simulink model "ME561FinalProjectSimulink_DiscreteNoFbOptimized_Stability"  (R2020a)
settings: Solver=ode5  StartTime=0.0  StopTime=800  FixedStep=0.01  RelTol=1e-3
values from neighbouring files (symbols this model uses):
  dB = 0.87    [ME561FinalProject.m]
  g = -9.81    [ME561FinalProject.m]
  humanSamplingTime = 0.01    [ME561FinalProject.m]
  JB = 66    [ME561FinalProject.m]
  KdDiscrete = K*Td/T    (= 19500)    [ME561FinalProject.m]
  KiDiscrete = K*T/Ti    (= 30)    [ME561FinalProject.m]
  Kn = 462    [ME561FinalProject.m]
  KpDiscrete = K - K*T/(2*Ti)    (= 435)    [ME561FinalProject.m]
  mB = 76    [ME561FinalProject.m]
  thetaRef = 0    [ME561FinalProject.m]
  timeNoise = 100    [ME561FinalProject.m]
libraries: simulink x1, simulink_extras x1
settings Model: Creator=jcferris  LastModifiedBy=jcferris

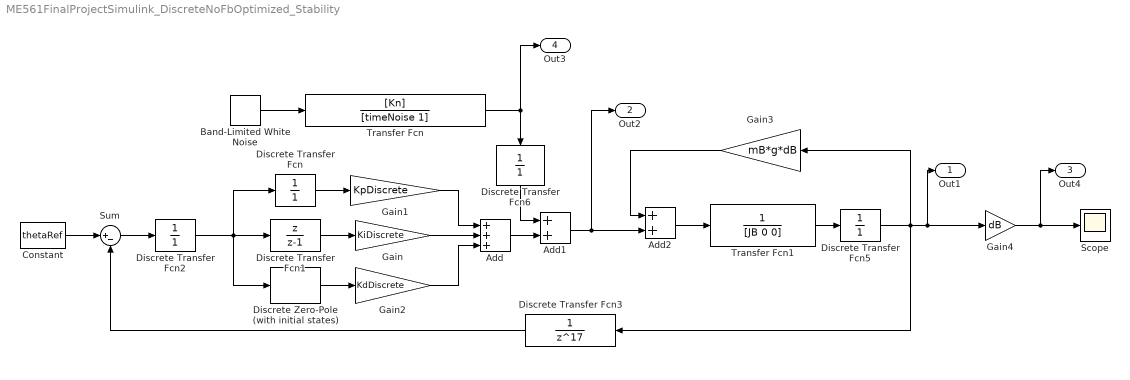
== system ME561FinalProjectSimulink_DiscreteNoFbOptimized_Stability ==
  Add : Sum  Inputs=+++
  Add1 : Sum
  Add2 : Sum
  Band-Limited White Noise : simulink/Sources/Band-Limited White Noise  Cov=[0.01]  Ts=0.01  seed=[23341]
  Constant : Constant  Value=thetaRef
  Discrete Transfer Fcn : DiscreteTransferFcn  Denominator=[1]
  Discrete Transfer Fcn1 : DiscreteTransferFcn  Numerator=[1 0]  Denominator=[1 -1]
  Discrete Transfer Fcn2 : DiscreteTransferFcn  Denominator=[1]  SampleTime=humanSamplingTime
  Discrete Transfer Fcn3 : DiscreteTransferFcn  Denominator=[1 0 0 0 0 0 0 0 0 0 0 0 0 0 0 0 0 0]
  Discrete Transfer Fcn5 : DiscreteTransferFcn  Denominator=[1]  SampleTime=humanSamplingTime
  Discrete Transfer Fcn6 : DiscreteTransferFcn  Denominator=[1]  SampleTime=humanSamplingTime
  Discrete Zero-Pole (with initial states) : simulink_extras/Additional Discrete/Discrete Zero-Pole (with initial states)  Z=[1]  P=[0]  K=[1]  X0=0  TS=-1
      settings: SourceProductBaseCode=SL
  Gain : Gain  Gain=KiDiscrete
  Gain1 : Gain  Gain=KpDiscrete
  Gain2 : Gain  Gain=KdDiscrete
  Gain3 : Gain  Gain=mB*g*dB
  Gain4 : Gain  Gain=dB
  Scope : Scope
  Sum : Sum  Inputs=|+-
  Transfer Fcn : TransferFcn  Numerator=[Kn]  Denominator=[timeNoise 1]
  Transfer Fcn1 : TransferFcn  Denominator=[JB 0 0]
  Out1 : Outport  SignalName=thetaStarOut
  Out2 : Outport  Port=2  SignalName=controlOutput
  Out4 : Outport  Port=3  SignalName=disp
  Out3 : Outport  Port=4  SignalName=disturb
  wires:
  Constant/1 -> Sum/1
  Gain/1 -> Add/2
  Gain1/1 -> Add/1
  Gain2/1 -> Add/3
  Add/1 -> Add1/2
  Add2/1 -> Transfer Fcn1/1
  Gain3/1 -> Add2/1
  Discrete Transfer Fcn3/1 -> Sum/2
  Gain4/1 -> Out4/1, Scope/1
  Add1/1 -> Add2/2, Out2/1
  Discrete Transfer Fcn1/1 -> Gain/1
  Discrete Zero-Pole (with initial states)/1 -> Gain2/1
  Discrete Transfer Fcn/1 -> Gain1/1
  Sum/1 -> Discrete Transfer Fcn2/1
  Discrete Transfer Fcn2/1 -> Discrete Transfer Fcn/1, Discrete Zero-Pole (with initial states)/1, Discrete Transfer Fcn1/1
  Discrete Transfer Fcn5/1 -> Discrete Transfer Fcn3/1, Out1/1, Gain4/1, Gain3/1
  Band-Limited White Noise/1 -> Transfer Fcn/1
  Transfer Fcn1/1 -> Discrete Transfer Fcn5/1
  Discrete Transfer Fcn6/1 -> Add1/1
  Transfer Fcn/1 -> Discrete Transfer Fcn6/1, Out3/1
